simulink model "PD"  (R2024b)
settings: Solver=VariableStepAuto  StartTime=0.0  StopTime=5  RelTol=1e-3
undefined symbols (not defined in the file): DiscIntNeverNeededParam
libraries: matrix_library x1
settings Model: Creator=prani  LastModifiedBy=prani

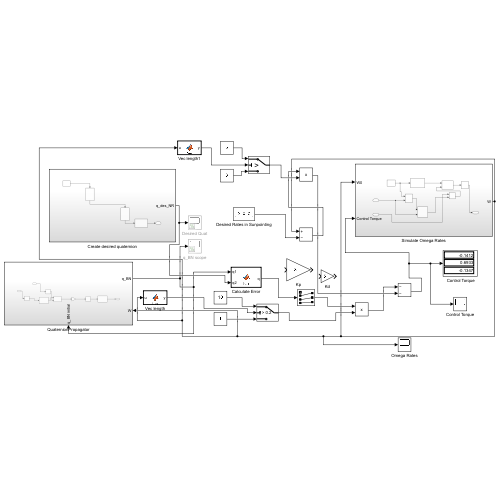
[thumbnail: Simulink's stored preview of the top-level diagram]
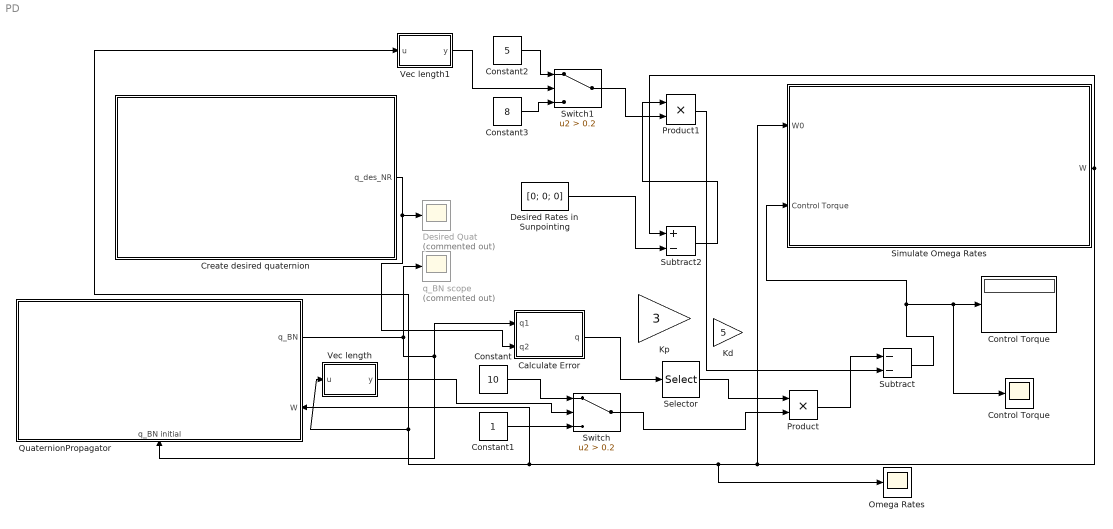
== system PD ==
  " Control Torque" : Display
  Calculate Error : MATLAB Function  TreatAsAtomicUnit=on
  Constant : Constant  Value=10
  Constant1 : Constant
  Constant2 : Constant  Value=5
  Constant3 : Constant  Value=8
  Control Torque : Scope
  Create desired quaternion : Subsystem
  Desired Quat : Scope  Commented=on
  Desired Rates in Sunpointing : Constant  Value=[0; 0; 0]
  Kd : Gain  Gain=5
  Kp : Gain  Gain=3
  Omega Rates : Scope
  Product : Product
  Product1 : Product
  QuaternionPropagator : Subsystem
      settings: PortSchema="{\"entries\":[{\"content\":{\"sides\":[{\"content\":{},\"type\":\"ConnectorPlacement.EquallySpacedRectSide\",\"uuid\":\"9e22cb63-f739-4def-bc16-8f5ac96da1b2\"},{\"content\":{\"connectorIds\":[\"Out1\",\"In2\"],\"side\":\"RIGHT\"},\"type\":\"ConnectorPlacement.EquallySpacedRectSide\",\"uuid\":\"185e8ae2-f047-4dfe-b4b8-b24ace8a5036\"},{\"content\":{\"side\":\"TOP\"},\"type\":\"ConnectorPlacement.EquallySpacedRectSide\",\"uuid\":\"aba5f04b-f2ef-4373-8d95-838bf2fc0f7e\"},{\"content\":{\"connectorIds\":[\"In1\"],\"side\":\"BOTTOM\"},\"type\":\"ConnectorPlacement.EquallySpacedRectSide\",\"uuid\":\"34d3ae2b-3f47-4699-99b9-a603dee72b74\"}]},\"type\":\"ConnectorPlacement.EquallySpacedConnector\",\"uuid\":\"020a8ac0-54fe-466e-8166-8e2d9bca8ffa\"}],\"packageUris\":[\"http://schema.mathworks.com/mf0/Connector/R2020b\"],\"version\":\"1.0\"}"
  Selector : Selector  InputPortWidth=4  IndexOptions=Index vector (dialog)  Indices=[2 : 4]  OutputSizes=1
  Simulate Omega Rates : Subsystem
  Subtract : Sum  Inputs=--
  Subtract2 : Sum  Inputs=+-
  Switch : Switch  Criteria=u2 > Threshold  Threshold=0.2  SaturateOnIntegerOverflow=off  InputSameDT=off
  Switch1 : Switch  Criteria=u2 > Threshold  Threshold=0.2  SaturateOnIntegerOverflow=off  InputSameDT=off
  Vec length : MATLAB Function  TreatAsAtomicUnit=on
  Vec length1 : MATLAB Function  TreatAsAtomicUnit=on
  q_BN scope : Scope  Commented=on
  wires:
  Subtract/1 -> Simulate Omega Rates/2(Control Torque), Control Torque/1, " Control Torque"/1
  Desired Rates in Sunpointing/1 -> Subtract2/2
  Simulate Omega Rates/1(W) -> Omega Rates/1, Vec length1/1(u), Vec length/1(u), QuaternionPropagator/2(W), Simulate Omega Rates/1(W0), Subtract2/1
  Create desired quaternion/1(q_des_NR) -> Calculate Error/2(q2), Desired Quat/1
  QuaternionPropagator/1(q_BN) -> QuaternionPropagator/1(q_BN initial), Calculate Error/1(q1), q_BN scope/1
  Vec length/1(y) -> Switch/2
  Switch/1 -> Product/2
  Calculate Error/1(q) -> Selector/1
  Vec length1/1(y) -> Switch1/2
  Constant2/1 -> Switch1/1
  Constant3/1 -> Switch1/3
  Switch1/1 -> Product1/2
  Subtract2/1 -> Product1/1
  Product1/1 -> Subtract/2
  Selector/1 -> Product/1
  Product/1 -> Subtract/1
  Constant1/1 -> Switch/3
  Constant/1 -> Switch/1

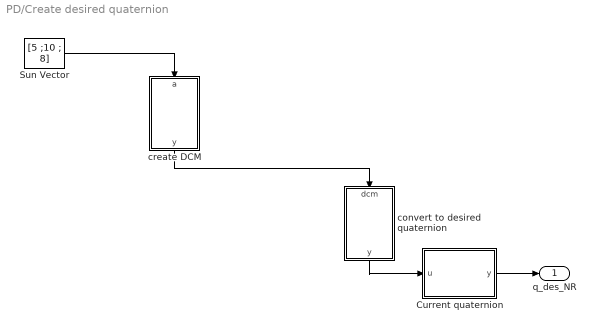
== system PD/Create desired quaternion ==
  Current quaternion : MATLAB Function  TreatAsAtomicUnit=on
  Sun Vector : Constant  Value=[5 ;10 ; 8]
  convert to desired quaternion : MATLAB Function  TreatAsAtomicUnit=on
  create DCM : MATLAB Function  TreatAsAtomicUnit=on
  q_des_NR : Outport
  wires:
  convert to desired quaternion/1(y) -> Current quaternion/1(u)
  Sun Vector/1 -> create DCM/1(a)
  create DCM/1(y) -> convert to desired quaternion/1(dcm)
  Current quaternion/1(y) -> q_des_NR/1

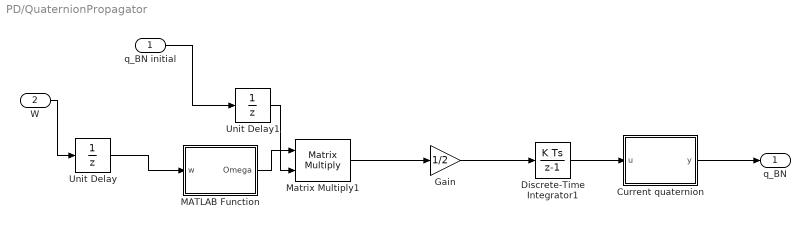
== system PD/QuaternionPropagator ==
  q_BN initial : Inport
  W : Inport  Port=2
  Current quaternion : MATLAB Function  TreatAsAtomicUnit=on
  Discrete-Time Integrator1 : DiscreteIntegrator  gainval=1  InitialCondition=[1; 0 ;0; 0]  SampleTime=0.1  ICPrevOutput=DiscIntNeverNeededParam  ICPrevScaledInput=DiscIntNeverNeededParam
  Gain : Gain  Gain=1/2
  MATLAB Function : MATLAB Function  TreatAsAtomicUnit=on
  Matrix Multiply1 : Product  Multiplication=Matrix(*)
  Unit Delay : UnitDelay  InitialCondition=[1; 1; 1]  SampleTime=-1  HasFrameUpgradeWarning=on
  Unit Delay1 : UnitDelay  InitialCondition=[1; 0; 0 ;0]  SampleTime=-1  HasFrameUpgradeWarning=on
  q_BN : Outport
  wires:
  Discrete-Time Integrator1/1 -> Current quaternion/1(u)
  Matrix Multiply1/1 -> Gain/1
  Current quaternion/1(y) -> q_BN/1
  Gain/1 -> Discrete-Time Integrator1/1
  MATLAB Function/1(Omega) -> Matrix Multiply1/1
  W/1 -> Unit Delay/1
  Unit Delay/1 -> MATLAB Function/1(w)
  Unit Delay1/1 -> Matrix Multiply1/2
  q_BN initial/1 -> Unit Delay1/1

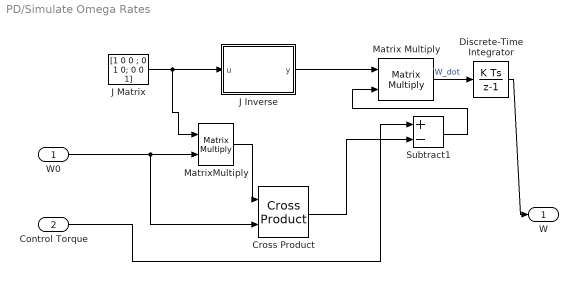
== system PD/Simulate Omega Rates ==
  W0 : Inport
  Control Torque : Inport  Port=2
  Cross Product : matrix_library/Cross Product
  Discrete-Time Integrator : DiscreteIntegrator  gainval=1  InitialCondition=[1; 1; 1]  SampleTime=0.1  ICPrevOutput=DiscIntNeverNeededParam  ICPrevScaledInput=DiscIntNeverNeededParam
  J Inverse : MATLAB Function  TreatAsAtomicUnit=on
  J Matrix : Constant  Value=[1 0 0 ; 0 1 0; 0 0 1]
  Matrix Multiply : Product  Multiplication=Matrix(*)
  MatrixMultiply : Product  Multiplication=Matrix(*)
  Subtract1 : Sum  Inputs=+-
  W : Outport
  wires:
  Matrix Multiply/1 -> Discrete-Time Integrator/1  "W_dot"
  Cross Product/1 -> Subtract1/2
  J Matrix/1 -> MatrixMultiply/1, J Inverse/1(u)
  MatrixMultiply/1 -> Cross Product/1
  J Inverse/1(y) -> Matrix Multiply/1
  Control Torque/1 -> Subtract1/1
  Subtract1/1 -> Matrix Multiply/2
  W0/1 -> Cross Product/2, MatrixMultiply/2
  Discrete-Time Integrator/1 -> W/1

== matlab function PD/Simulate Omega Rates/J Inverse ==
  data: u input; y output
function y = fcn(u)

y = inv(u);

== matlab function PD/QuaternionPropagator/Current quaternion ==
  data: u input; y output
function y = fcn(u)

y = u/norm(u);

== matlab function PD/Create desired quaternion/create DCM ==
  data: a input; y output
function y = fcn(a)

unitx = [1 0 0];
unity = [0 1 0];
b=cross(a, unitx);
if dot(a,b)<1e6
b= cross(a,unity);
end

c = cross(a,b);
y = [ a(:), b(:), c(:)];
end

== matlab function PD/Create desired quaternion/convert to desired quaternion ==
  data: dcm input; y output
function y = fcn(dcm)
%  DCM2QUAT Convert direction cosine matrix to quaternion.
%   Q = DCM2QUAT( DCM ) calculates the quaternion, Q, for given direction
%   cosine matrix, DCM. 
% 
%   Q = DCM2QUAT( DCM, ACTION ) uses ACTION for error handling during
%   rotation matrix validation. 
%
%   Q = DCM2QUAT( DCM, ACTION, TOL ) uses TOL as a relative error tolerance
%   for rotation matrix validation. 
%   eps(2).
%
% Inputs:
%   DCM    :3-by-3-by-M matrix containing M orthogonal direction cosine matrices.
%           DCM performs the coordinate transformation from inertial axes to body axes. 
%   ACTION :Scalar string specifying the action to take if the DCM is invalid.
%           Valid directon cosine matricies are orthogonal and proper:
%           transpose(DCM) * DCM == 1 +/- TOL
%           det(DCM) == 1 +/- TOL
%           ACTION must be one of the following:
%             'Error'
%             'Warning'
%             'None'
%           Default is 'None'.
%   TOL    :Scalar numeric specifying the relative tolerance for rotation matrix validation.
%           The tolerance is used for validating the direction cosine matricies.
%           Default value is eps(2).
%
% Outputs:
%   Q :M-by-4 matrix of quaternions vectors. Q has its scalar number as the first
%      column.
%
% Examples:
%   Determine the quaternion from a direction cosine matrix:
%      dcm = [0 1 0; 1 0 0; 0 0 -1];
%      q = dcm2quat(dcm)
%
%   Determine the quaternions from multiple direction cosine matrices:
%      dcm        = [ 0 1 0; 1 0 0; 0 0 -1]; 
%      dcm(:,:,2) = [ 0.4330    0.2500   -0.8660; ...
%                     0.1768    0.9186    0.3536; ...
%                     0.8839   -0.3062    0.3536];
%      q = dcm2quat(dcm)
%
%   Determine the quaternion from a direction cosine matrix with a specified
%   action and tolerance:
%      dcm = [0 1 0; 1 0 0; 0 0 -1];
%      q = dcm2quat(dcm, 'warning', 0.01)
%
%   See also ANGLE2DCM, DCM2ANGLE, QUAT2DCM, QUAT2ANGLE, ANGLE2QUAT.

%   Copyright 2000-2020 The MathWorks, Inc.

q =[1 0 0 0];
for i = size(dcm,3):-1:1

    q(i,4) =  0; 
    
    tr = trace(dcm(:,:,i));

    if (tr > 0)
        sqtrp1 = sqrt( tr + 1.0 );
        
        q(i,1) = 0.5*sqtrp1; 
        q(i,2) = (dcm(2, 3, i) - dcm(3, 2, i))/(2.0*sqtrp1);
        q(i,3) = (dcm(3, 1, i) - dcm(1, 3, i))/(2.0*sqtrp1); 
        q(i,4) = (dcm(1, 2, i) - dcm(2, 1, i))/(2.0*sqtrp1); 
    else
        d = diag(dcm(:,:,i));
        if ((d(2) > d(1)) && (d(2) > d(3)))
            % max value at dcm(2,2,i)
            sqdip1 = sqrt(d(2) - d(1) - d(3) + 1.0 );
            
            q(i,3) = 0.5*sqdip1; 
            
            if ( sqdip1 ~= 0 )
                sqdip1 = 0.5/sqdip1;
            end
            
            q(i,1) = (dcm(3, 1, i) - dcm(1, 3, i))*sqdip1; 
            q(i,2) = (dcm(1, 2, i) + dcm(2, 1, i))*sqdip1; 
            q(i,4) = (dcm(2, 3, i) + dcm(3, 2, i))*sqdip1; 
        elseif (d(3) > d(1))
            % max value at dcm(3,3,i)
            sqdip1 = sqrt(d(3) - d(1) - d(2) + 1.0 );
            
            q(i,4) = 0.5*sqdip1; 
            
            if ( sqdip1 ~= 0 )
                sqdip1 = 0.5/sqdip1;
            end
            
            q(i,1) = (dcm(1, 2, i) - dcm(2, 1, i))*sqdip1;
            q(i,2) = (dcm(3, 1, i) + dcm(1, 3, i))*sqdip1; 
            q(i,3) = (dcm(2, 3, i) + dcm(3, 2, i))*sqdip1; 
        else
            % max value at dcm(1,1,i)
            sqdip1 = sqrt(d(1) - d(2) - d(3) + 1.0 );
            
            q(i,2) = 0.5*sqdip1; 
            
            if ( sqdip1 ~= 0 )
                sqdip1 = 0.5/sqdip1;
            end
            
            q(i,1) = (dcm(2, 3, i) - dcm(3, 2, i))*sqdip1; 
            q(i,3) = (dcm(1, 2, i) + dcm(2, 1, i))*sqdip1; 
            q(i,4) = (dcm(3, 1, i) + dcm(1, 3, i))*sqdip1; 
        end
    end
end
y=transpose(q);
end

== matlab function PD/Calculate Error ==
  data: q1 input; q output; q2 input
function q = fcn(q1, q2)

    w1 = q1(1); x1 = q1(2); y1 = q1(3); z1 = q1(4);
    w2 = q2(1); x2 = q2(2); y2 = q2(3); z2 = q2(4);

    w = w1*w2 - x1*x2 - y1*y2 - z1*z2;
    x = w1*x2 + x1*w2 + y1*z2 - z1*y2;
    y = w1*y2 - x1*z2 + y1*w2 + z1*x2;
    z = w1*z2 + x1*y2 - y1*x2 + z1*w2;

    q = [w; x; y; z];
end

== matlab function PD/Create desired quaternion/Current quaternion ==
  data: u input; y output
function y = fcn(u)

y = u/norm(u);

== matlab function PD/Vec length ==
  data: u input; y output
function y = fcn(u)

y = sqrt(u(1)^2+u(2)^2+u(3)^2);

== matlab function PD/Vec length1 ==
  data: u input; y output
function y = fcn(u)

y = sqrt(u(1)^2+u(2)^2+u(3)^2);

== matlab function PD/QuaternionPropagator/MATLAB Function ==
  data: w input; Omega output
function Omega = fcn(w)

wx = w(1); wy = w(2); wz = w(3);

Omega = [ 0   -wx  -wy  -wz;
          wx   0    wz  -wy;
          wy  -wz   0    wx;
          wz   wy  -wx   0  ];
